simulink model "deadzone_sim"  (R2015a)
settings: Solver=ode45  StartTime=0.0  StopTime=120  RelTol=1e-3
settings Model: SimulationMode=accelerator  Creator=jinkale  LastModifiedBy=jinkale

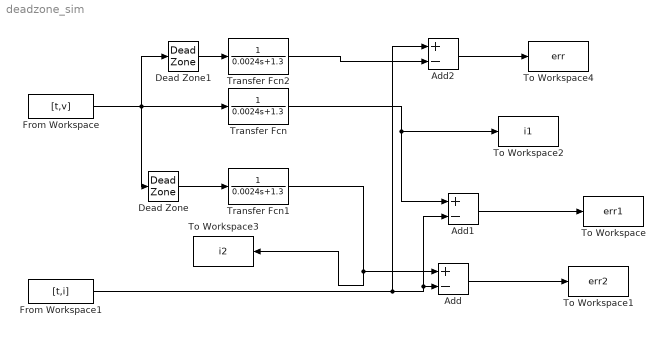
== system deadzone_sim ==
  Add : Sum  Inputs=+-
  Add1 : Sum  Inputs=+-
  Add2 : Sum  Inputs=+-
  Dead Zone : DeadZone  LowerValue=-0.4621  UpperValue=0.4621  SaturateOnIntegerOverflow=on
  Dead Zone1 : DeadZone  LowerValue=-0.4621  UpperValue=0.4621  SaturateOnIntegerOverflow=on
  From Workspace : FromWorkspace  VariableName=[t,v]  SampleTime=0
  From Workspace1 : FromWorkspace  VariableName=[t,i]  SampleTime=0
  To Workspace : ToWorkspace  VariableName=err1  SaveFormat=Timeseries  SampleTime=1/200
  To Workspace1 : ToWorkspace  VariableName=err2  SaveFormat=Timeseries  SampleTime=1/200
  To Workspace2 : ToWorkspace  VariableName=i1  SaveFormat=Timeseries  SampleTime=1/200
  To Workspace3 : ToWorkspace  VariableName=i2  SaveFormat=Timeseries  SampleTime=1/200
  To Workspace4 : ToWorkspace  VariableName=err  SaveFormat=Timeseries  SampleTime=1/200
  Transfer Fcn : TransferFcn  Denominator=[0.0024 1.3]
  Transfer Fcn1 : TransferFcn  Denominator=[0.0024 1.3]
  Transfer Fcn2 : TransferFcn  Denominator=[0.0024 1.3]
  wires:
  From Workspace/1 -> Dead Zone1/1, Dead Zone/1, Transfer Fcn/1
  Dead Zone/1 -> Transfer Fcn1/1
  From Workspace1/1 -> Add2/1, Add1/2, Add/2
  Transfer Fcn/1 -> Add1/1, To Workspace2/1
  Transfer Fcn1/1 -> To Workspace3/1, Add/1
  Add1/1 -> To Workspace/1
  Add/1 -> To Workspace1/1
  Dead Zone1/1 -> Transfer Fcn2/1
  Add2/1 -> To Workspace4/1
  Transfer Fcn2/1 -> Add2/2
